simulink model "im_with_m1act_damp"  (R2022b)
settings: Solver=FixedStepAuto  StartTime=0.0  StopTime=5  FixedStep=FEM_Ts  MaxStep=FEM_Ts  RelTol=1e-2
InitFcn:
  | %
  | % Initialization callback function
  | %
  | 
  | try
  |    fprintf('\nGMT IMS version (%s)!\n',simulink_fname );
  | 
  |    % Get Simulink model directory
  |    [filepath,name,ext] = fileparts(which(bdroot));
  | 
  |    if ~strcmp(filepath,pwd)
  |       fprintf('\nChanging current directory to \n %s \n',filepath);
  |       cd(filepath);
  |    end
  | 
  |    %
  |  if(osim.bpless_wl)
  |     fprintf('Generating bumpless wind load time series\n');
  |  end
  | catch
  |    warning('Running the InitFcn from puSimulate script');
  | end
values from neighbouring files (symbols this model uses):
  a_max = 250e-6    (= 0.00025)    [load_im_with_m1act_damp.m]    (also in load_m1hp_cpp_demo.m)
  b = B(:,in)*m1sys{seg}.Kbal    [evalM1ofl_act_damp.m]
  c = [Upsilon*C(out0,:);     C(out1a,:)-C(out1b,:);     C(out2,:)]    [evalM1ofl_act_damp.m]
  CS_Upsilon = [0 0 1 3.6925 1.6038 0 0 0 1 0.99769 3.9002 0 ... (1836 elements, 6x306)]    [CS_SupportActuatorArrayConfig.mat]
  delta_sim = 1e-3    (= 0.001)    [load_im_with_m1act_damp.m]    (also in load_m1hp_cpp_demo.m)
  drv_delay = ceil(mount.delay/FEM_Ts)    [load_im_with_m1act_damp.m]    (also in load_m1hp_cpp_demo.m)
  FEM_Ts = 1/1e3    (= 0.001)    [load_im_with_m1act_damp.m]    (also in load_m1hp_cpp_demo.m)
  Hdrive_d = c2d(o.Hdrive(1,1), FEM_Ts, 'tustin')    [load_im_with_m1act_damp.m]    (also in load_m1hp_cpp_demo.m)
  m1_act_lin_d = osim.m1act_damp*1800    [load_im_with_m1act_damp.m]
  m1_act_quad_d = 9000    [load_im_with_m1act_damp.m]
  m1sys = ovr_ofl_crtl(m1sys,seg)    [evalM1ofl_act_damp.m]    (also in load_im_with_m1act_damp.m = ovr_ofl_crtl(m1sys))
  M_cs_abc2xyz = M_cs_abc2xyzT'    [calc_ort2cylTs.m]
  M_oa_abc2xyz = M_oa_abc2xyzT'    [calc_ort2cylTs.m]
  o = fun_confBase(oTest)    [load_im_with_m1act_damp.m]    (also in load_m1hp_cpp_demo.m)
  OA_Upsilon = [1 0 0 0 -0.308856 0.000749419 0 1 0 0.308856 0 0.776768 ... (2010 elements, 6x335)]    [OA_SupportActuatorArrayConfig.mat]
  PG = zeros(length(om2),6)    [load_im_with_m1act_damp.m]    (also in load_m1hp_cpp_demo.m)
  phiB = inputs2ModalF(mode_ind_vec,indDesInputs)    [load_im_with_m1act_damp.m]    (also in load_m1hp_cpp_demo.m)
  phiC = modalDisp2Outputs(indDesOutputs,mode_ind_vec)    [load_im_with_m1act_damp.m]    (also in load_m1hp_cpp_demo.m)
  phiCvel = modalDisp2Outputs(ind_M1act_vel,mode_ind_vec)    [load_im_with_m1act_damp.m]
  Psi_ss = gainMatrix(indDesOutputs,indDesInputs) - K_ss    [load_im_with_m1act_damp.m]    (also in load_m1hp_cpp_demo.m)
  t_gd = 0*0.5    (= 0)    [load_im_with_m1act_damp.m]    (also in load_m1hp_cpp_demo.m)
  t_gd_v = 0*t_gd    (= 0)    [load_im_with_m1act_damp.m]    (also in load_m1hp_cpp_demo.m)
  Tcmd = 12    [load_im_with_m1act_damp.m]    (also in load_m1hp_cpp_demo.m)
  v0 = 0    [load_im_with_m1act_damp.m]    (also in load_m1hp_cpp_demo.m)
  v_max = 50e-6    (= 5e-05)    [load_im_with_m1act_damp.m]    (also in load_m1hp_cpp_demo.m)
  x0 = 0    [load_im_with_m1act_damp.m]    (also in load_m1hp_cpp_demo.m)
  x0_f = xf(end,:)    [load_im_with_m1act_damp.m]    (also in load_m1hp_cpp_demo.m)
undefined symbols (not defined in the file or in its folder): a, A_f, az, az_ff_en, B_f, C_f, D_f, DiscIntNeverNeededParam, el, gir, M_cs_xyz2abc, M_oa_xyz2abc, magnitude, mount, osim
libraries: simulink x9, ims_block_library x7, simulink_extras x2
(part 2 of 3)

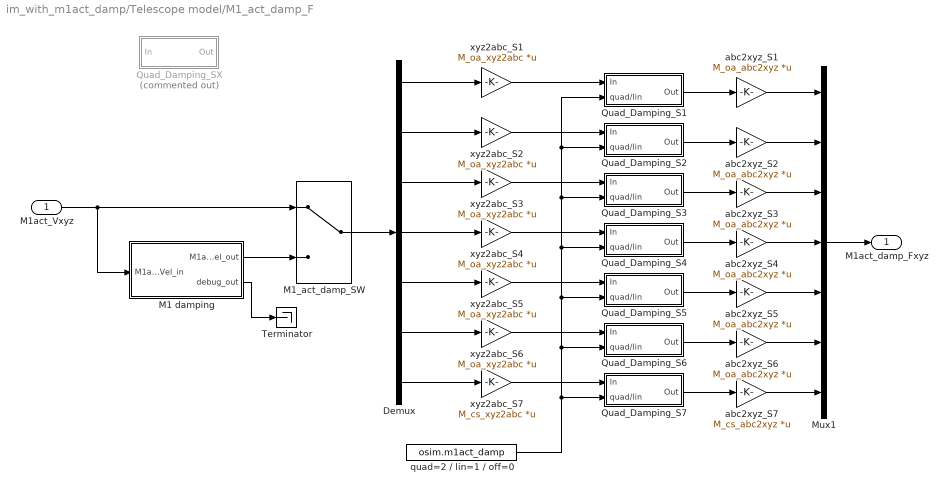
== system im_with_m1act_damp/Telescope model/M1_act_damp_F ==
  M1act_Vxyz : Inport
  Demux : Demux  Outputs=[335,335,335,335,335,335,306]
  M1 damping : Subsystem
  M1_act_damp_SW : ManualSwitch
  Mux1 : Mux  Inputs=[335,335,335,335,335,335,306]
  Quad_Damping_S1 : Subsystem
  Quad_Damping_S2 : Subsystem
  Quad_Damping_S3 : Subsystem
  Quad_Damping_S4 : Subsystem
  Quad_Damping_S5 : Subsystem
  Quad_Damping_S6 : Subsystem
  Quad_Damping_S7 : Subsystem
  Quad_Damping_SX : Subsystem  Commented=on
  Terminator : Terminator
  abc2xyz_S{1..6} (6 alike) : Gain  Gain=M_oa_abc2xyz  Multiplication=Matrix(K*u) (u vector)
  abc2xyz_S7 : Gain  Gain=M_cs_abc2xyz  Multiplication=Matrix(K*u) (u vector)
  quad=2 / lin=1 / off=0 : Constant  Value=osim.m1act_damp
  xyz2abc_S{1..6} (6 alike) : Gain  Gain=M_oa_xyz2abc  Multiplication=Matrix(K*u) (u vector)
  xyz2abc_S7 : Gain  Gain=M_cs_xyz2abc  Multiplication=Matrix(K*u) (u vector)
  M1act_damp_Fxyz : Outport
  wires:
  M1 damping/1(M1act_Vel_out) -> M1_act_damp_SW/2
  Mux1/1 -> M1act_damp_Fxyz/1
  M1act_Vxyz/1 -> M1 damping/1(M1act_Vel_in), M1_act_damp_SW/1
  M1 damping/2(debug_out) -> Terminator/1
  Quad_Damping_S1/1(Out) -> abc2xyz_S1/1
  xyz2abc_S2/1 -> Quad_Damping_S2/1(In)
  abc2xyz_S4/1 -> Mux1/4
  Demux/2 -> xyz2abc_S2/1
  abc2xyz_S7/1 -> Mux1/7
  Demux/5 -> xyz2abc_S5/1
  Quad_Damping_S7/1(Out) -> abc2xyz_S7/1
  Demux/7 -> xyz2abc_S7/1
  abc2xyz_S3/1 -> Mux1/3
  xyz2abc_S5/1 -> Quad_Damping_S5/1(In)
  M1_act_damp_SW/1 -> Demux/1
  Quad_Damping_S6/1(Out) -> abc2xyz_S6/1
  abc2xyz_S1/1 -> Mux1/1
  xyz2abc_S3/1 -> Quad_Damping_S3/1(In)
  Quad_Damping_S5/1(Out) -> abc2xyz_S5/1
  Demux/3 -> xyz2abc_S3/1
  abc2xyz_S2/1 -> Mux1/2
  Quad_Damping_S4/1(Out) -> abc2xyz_S4/1
  Demux/1 -> xyz2abc_S1/1
  xyz2abc_S7/1 -> Quad_Damping_S7/1(In)
  Demux/4 -> xyz2abc_S4/1
  Demux/6 -> xyz2abc_S6/1
  Quad_Damping_S2/1(Out) -> abc2xyz_S2/1
  xyz2abc_S4/1 -> Quad_Damping_S4/1(In)
  xyz2abc_S1/1 -> Quad_Damping_S1/1(In)
  abc2xyz_S6/1 -> Mux1/6
  xyz2abc_S6/1 -> Quad_Damping_S6/1(In)
  Quad_Damping_S3/1(Out) -> abc2xyz_S3/1
  abc2xyz_S5/1 -> Mux1/5
  quad=2 / lin=1 / off=0/1 -> Quad_Damping_S6/2(quad/lin), Quad_Damping_S2/2(quad/lin), Quad_Damping_S1/2(quad/lin), Quad_Damping_S3/2(quad/lin), Quad_Damping_S4/2(quad/lin), Quad_Damping_S5/2(quad/lin), Quad_Damping_S7/2(quad/lin)

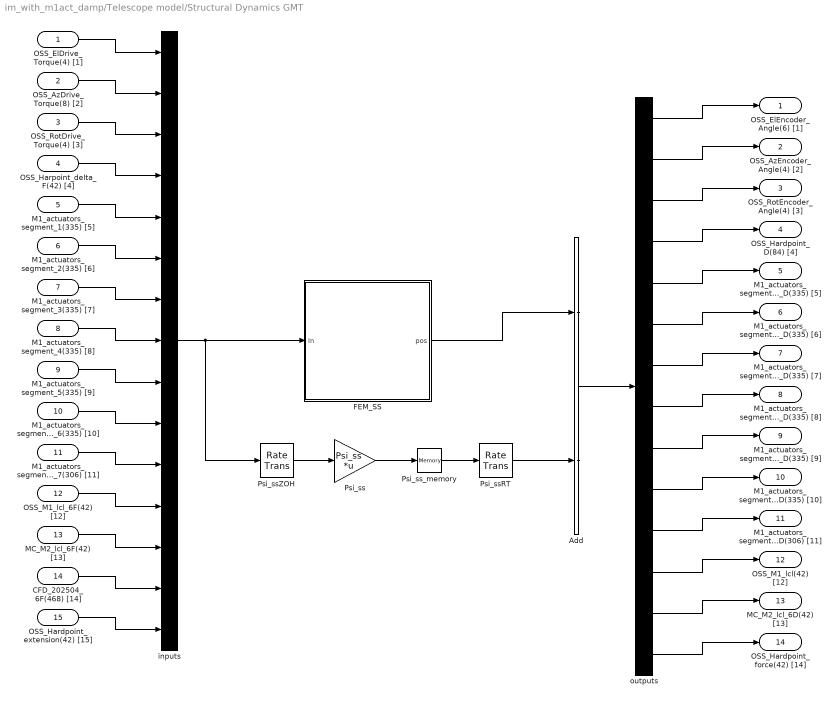
== system im_with_m1act_damp/Telescope model/Structural Dynamics GMT ==
  OSS_ElDrive_Torque(4) [1] : Inport  PortDimensions=4
  OSS_AzDrive_Torque(8) [2] : Inport  Port=2  PortDimensions=8
  OSS_RotDrive_Torque(4) [3] : Inport  Port=3  PortDimensions=4
  OSS_Harpoint_delta_F(42) [4] : Inport  Port=4  PortDimensions=42
  M1_actuators_segment_1(335) [5] : Inport  Port=5  PortDimensions=335
  M1_actuators_segment_2(335) [6] : Inport  Port=6  PortDimensions=335
  M1_actuators_segment_3(335) [7] : Inport  Port=7  PortDimensions=335
  M1_actuators_segment_4(335) [8] : Inport  Port=8  PortDimensions=335
  M1_actuators_segment_5(335) [9] : Inport  Port=9  PortDimensions=335
  M1_actuators_segment_6(335) [10] : Inport  Port=10  PortDimensions=335
  M1_actuators_segment_7(306) [11] : Inport  Port=11  PortDimensions=306
  OSS_M1_lcl_6F(42) [12] : Inport  Port=12  PortDimensions=42
  MC_M2_lcl_6F(42) [13] : Inport  Port=13  PortDimensions=42
  CFD_202504_6F(468) [14] : Inport  Port=14  PortDimensions=468
  OSS_Hardpoint_extension(42) [15] : Inport  Port=15  PortDimensions=42
  Add : Sum
  FEM_SS : Subsystem
  Psi_ss : Gain  Gain=Psi_ss  Multiplication=Matrix(K*u) (u vector)
  Psi_ssRT : RateTransition  Integrity=off  OutPortSampleTimeOpt=Inherit
  Psi_ssZOH : RateTransition  Integrity=off  OutPortSampleTime=Psi_ssTs
  Psi_ss_memory : Memory  InitialCondition=zeros(size(phiC,1),1)  InheritSampleTime=on  LinearizeAsDelay=on
  inputs : Mux  Inputs=modelMuxDims
  outputs : Demux  Outputs=modelDemuxDims
  OSS_ElEncoder_Angle(6) [1] : Outport  PortDimensions=6
  OSS_AzEncoder_Angle(4) [2] : Outport  Port=2  PortDimensions=4
  OSS_RotEncoder_Angle(4) [3] : Outport  Port=3  PortDimensions=4
  OSS_Hardpoint_D(84) [4] : Outport  Port=4  PortDimensions=84
  M1_actuators_segment_1_D(335) [5] : Outport  Port=5  PortDimensions=335
  M1_actuators_segment_2_D(335) [6] : Outport  Port=6  PortDimensions=335
  M1_actuators_segment_3_D(335) [7] : Outport  Port=7  PortDimensions=335
  M1_actuators_segment_4_D(335) [8] : Outport  Port=8  PortDimensions=335
  M1_actuators_segment_5_D(335) [9] : Outport  Port=9  PortDimensions=335
  M1_actuators_segment_6_D(335) [10] : Outport  Port=10  PortDimensions=335
  M1_actuators_segment_7_D(306) [11] : Outport  Port=11  PortDimensions=306
  OSS_M1_lcl(42) [12] : Outport  Port=12  PortDimensions=42
  MC_M2_lcl_6D(42) [13] : Outport  Port=13  PortDimensions=42
  OSS_Hardpoint_force(42) [14] : Outport  Port=14  PortDimensions=42
  wires:
  outputs/14 -> OSS_Hardpoint_force(42) [14]/1
  outputs/13 -> MC_M2_lcl_6D(42) [13]/1
  outputs/12 -> OSS_M1_lcl(42) [12]/1
  outputs/11 -> M1_actuators_segment_7_D(306) [11]/1
  outputs/10 -> M1_actuators_segment_6_D(335) [10]/1
  outputs/9 -> M1_actuators_segment_5_D(335) [9]/1
  outputs/8 -> M1_actuators_segment_4_D(335) [8]/1
  outputs/7 -> M1_actuators_segment_3_D(335) [7]/1
  outputs/6 -> M1_actuators_segment_2_D(335) [6]/1
  outputs/5 -> M1_actuators_segment_1_D(335) [5]/1
  outputs/4 -> OSS_Hardpoint_D(84) [4]/1
  outputs/3 -> OSS_RotEncoder_Angle(4) [3]/1
  outputs/2 -> OSS_AzEncoder_Angle(4) [2]/1
  outputs/1 -> OSS_ElEncoder_Angle(6) [1]/1
  OSS_Hardpoint_extension(42) [15]/1 -> inputs/15
  CFD_202504_6F(468) [14]/1 -> inputs/14
  MC_M2_lcl_6F(42) [13]/1 -> inputs/13
  OSS_M1_lcl_6F(42) [12]/1 -> inputs/12
  M1_actuators_segment_7(306) [11]/1 -> inputs/11
  M1_actuators_segment_6(335) [10]/1 -> inputs/10
  M1_actuators_segment_5(335) [9]/1 -> inputs/9
  M1_actuators_segment_4(335) [8]/1 -> inputs/8
  M1_actuators_segment_3(335) [7]/1 -> inputs/7
  M1_actuators_segment_2(335) [6]/1 -> inputs/6
  M1_actuators_segment_1(335) [5]/1 -> inputs/5
  OSS_Harpoint_delta_F(42) [4]/1 -> inputs/4
  OSS_RotDrive_Torque(4) [3]/1 -> inputs/3
  OSS_AzDrive_Torque(8) [2]/1 -> inputs/2
  OSS_ElDrive_Torque(4) [1]/1 -> inputs/1
  Psi_ssZOH/1 -> Psi_ss/1
  Psi_ss_memory/1 -> Psi_ssRT/1
  Psi_ssRT/1 -> Add/2
  inputs/1 -> Psi_ssZOH/1, FEM_SS/1(In)
  FEM_SS/1(pos) -> Add/1
  Psi_ss/1 -> Psi_ss_memory/1
  Add/1 -> outputs/1

== system im_with_m1act_damp/Wind Loads/Sigmoid ==
  Add : Sum  Inputs=+-
  Add1 : Sum
  Clock : Clock
  Constant : Constant  Value=0.75
  CteOne : Constant
  Gain : Gain  Gain=-5
  Math Function : Math  SignedPower=on
  Reciprocal Function : Math  Operator=reciprocal  SignedPower=on
  Sqr Function : Math  Operator=square  SignedPower=on
  s : Outport
  wires:
  Sqr Function/1 -> Reciprocal Function/1
  Math Function/1 -> Add1/2
  Gain/1 -> Math Function/1
  Add/1 -> Gain/1
  Clock/1 -> Add/1
  Constant/1 -> Add/2
  Add1/1 -> Sqr Function/1
  CteOne/1 -> Add1/1
  Reciprocal Function/1 -> s/1

== system im_with_m1act_damp/M1 CPP/cmd_pre_proc/Bessel filter ==
  pos_vec : Inport  Partition=on  PartitionDimension=1  PartitionWidth=1  PartitionOffset=0
  vel_vec : Inport  Port=2  Partition=on  PartitionDimension=1  PartitionWidth=1  PartitionOffset=0
  acc_vec : Inport  Port=3  Partition=on  PartitionDimension=1  PartitionWidth=1  PartitionOffset=0
  For Each : ForEach  DisableCoverage=on  SpecifiedNumIters=n_in
  Jerk-limitation : Subsystem
  pos_f_vec : Outport  ConcatenationDimension=1
  vel_f_vec : Outport  Port=2  ConcatenationDimension=1
  acc_f_vec : Outport  Port=3  ConcatenationDimension=1
  wires:
  vel_vec/1 -> Jerk-limitation/2(vel)
  Jerk-limitation/3(pos_f) -> pos_f_vec/1
  Jerk-limitation/2(vel_f) -> vel_f_vec/1
  Jerk-limitation/1(acc_f) -> acc_f_vec/1
  pos_vec/1 -> Jerk-limitation/3(pos)
  acc_vec/1 -> Jerk-limitation/1(acc)

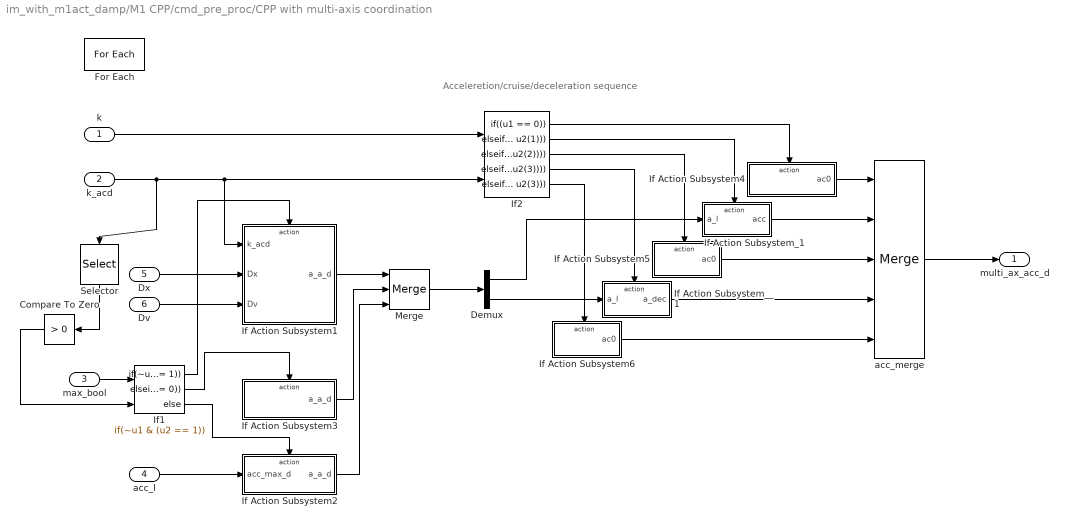
== system im_with_m1act_damp/M1 CPP/cmd_pre_proc/CPP with multi-axis coordination ==
  note: Acceleretion/cruise/deceleration sequence
  k : Inport
  k_acd : Inport  Port=2
  max_bool : Inport  Port=3  Partition=on  PartitionDimension=1  PartitionWidth=1  PartitionOffset=0
  acc_l : Inport  Port=4  Partition=on  PartitionDimension=1  PartitionWidth=1  PartitionOffset=0
  Dx : Inport  Port=5  Partition=on  PartitionDimension=1  PartitionWidth=1  PartitionOffset=0
  Dv : Inport  Port=6  Partition=on  PartitionDimension=1  PartitionWidth=1  PartitionOffset=0
  Compare To Zero : simulink/Logic and Bit Operations/Compare To Zero  relop=>  OutDataTypeStr=boolean
  Demux : Demux  Outputs=2
  For Each : ForEach  DisableCoverage=on
  If Action Subsystem1 : Subsystem  TreatAsAtomicUnit=on
  If Action Subsystem2 : Subsystem  TreatAsAtomicUnit=on
  If Action Subsystem3 : Subsystem  TreatAsAtomicUnit=on
  If Action Subsystem4 : Subsystem  TreatAsAtomicUnit=on
  If Action Subsystem5 : Subsystem  TreatAsAtomicUnit=on
  If Action Subsystem6 : Subsystem  TreatAsAtomicUnit=on
  If Action Subsystem_1 : Subsystem  TreatAsAtomicUnit=on
  If Action Subsystem__1 : Subsystem  TreatAsAtomicUnit=on
  If1 : If  NumInputs=2  IfExpression=~u1 & (u2 == 1)  ElseIfExpressions=~u1 & (u2 == 0)
  If2 : If  NumInputs=2  IfExpression=(u1 == 0)  ElseIfExpressions=(u1 <= u2(1)), ((u1 > u2(1)) & (u1 <= u2(2))), ((u1 > u2(2)) & (u1 <= u2(3))), (u1 > u2(3))  ShowElse=off
  Merge : Merge  Inputs=3
  Selector : Selector  InputPortWidth=3  IndexOptions=Index vector (dialog)  Indices=[3]  OutputSizes=1
  acc_merge : Merge  Inputs=5  InitialOutput=0
  multi_ax_acc_d : Outport  ConcatenationDimension=1
  wires:
  acc_merge/1 -> multi_ax_acc_d/1
  k/1 -> If2/1
  max_bool/1 -> If1/1
  If1/1 -> If Action Subsystem1/Action
  If1/3 -> If Action Subsystem2/Action
  acc_l/1 -> If Action Subsystem2/1(acc_max_d)
  If Action Subsystem2/1(a_a_d) -> Merge/3
  If Action Subsystem1/1(a_a_d) -> Merge/1
  Merge/1 -> Demux/1
  Dx/1 -> If Action Subsystem1/2(Dx)
  Dv/1 -> If Action Subsystem1/3(Dv)
  If Action Subsystem3/1(a_a_d) -> Merge/2
  Selector/1 -> Compare To Zero/1
  If1/2 -> If Action Subsystem3/Action
  Compare To Zero/1 -> If1/2
  If Action Subsystem5/1(ac0) -> acc_merge/3
  If2/1 -> If Action Subsystem4/Action
  Demux/2 -> If Action Subsystem__1/1(a_l)
  If Action Subsystem4/1(ac0) -> acc_merge/1
  If2/3 -> If Action Subsystem5/Action
  If2/4 -> If Action Subsystem__1/Action
  If Action Subsystem__1/1(a_dec) -> acc_merge/4
  If2/2 -> If Action Subsystem_1/Action
  If Action Subsystem_1/1(acc) -> acc_merge/2
  Demux/1 -> If Action Subsystem_1/1(a_l)
  If2/5 -> If Action Subsystem6/Action
  If Action Subsystem6/1(ac0) -> acc_merge/5
  k_acd/1 -> If2/2, If Action Subsystem1/1(k_acd), Selector/1

== system im_with_m1act_damp/M1 CPP/cmd_pre_proc/CPP with multi-axis coordination1 ==
  k : Inport
  k_acd : Inport  Port=2
  Demux1 : Demux  Outputs=3
  Dk_merge : Merge  Inputs=4  InitialOutput=0
  If Action Subsystem : Subsystem  TreatAsAtomicUnit=on
  If Action Subsystem1 : Subsystem  TreatAsAtomicUnit=on
  If Action Subsystem6 : Subsystem  TreatAsAtomicUnit=on
  If Action Subsystem__1 : Subsystem  TreatAsAtomicUnit=on
  If2 : If  NumInputs=2  IfExpression=(u1 == 0) | (u1 <= u2(1))  ElseIfExpressions=((u1 > u2(1)) & (u1 <= u2(2))), ((u1 > u2(2)) & (u1 <= u2(3))), (u1 > u2(3))  ShowElse=off
  Dk : Outport
  wires:
  k_acd/1 -> If2/2, Demux1/1
  k/1 -> If2/1
  Demux1/3 -> If Action Subsystem6/1(t_acd)
  If Action Subsystem__1/1(Dk) -> Dk_merge/3
  Demux1/1 -> If Action Subsystem1/1(t_a)
  If2/1 -> If Action Subsystem/Action
  If Action Subsystem/1(Dk) -> Dk_merge/1
  Demux1/2 -> If Action Subsystem__1/1(t_ac)
  If Action Subsystem1/1(Dk) -> Dk_merge/2
  If Action Subsystem6/1(Dk) -> Dk_merge/4
  Dk_merge/1 -> Dk/1
  If2/2 -> If Action Subsystem1/Action
  If2/3 -> If Action Subsystem__1/Action
  If2/4 -> If Action Subsystem6/Action

== system im_with_m1act_damp/M1 CPP/cmd_pre_proc/Motion equations ==
  acc_d : Inport  Partition=on  PartitionDimension=1  PartitionWidth=1  PartitionOffset=0
  k : Inport  Port=2
  Dk : Inport  Port=3
  Add : Sum  Inputs=+++
  Compare To Constant : simulink/Logic and Bit Operations/Compare To Constant  relop===  const=0  OutDataTypeStr=boolean
  Constant : Constant  Value=v0
  Detect Change : simulink/Logic and Bit Operations/Detect Change  vinit=0  OutDataTypeStr=boolean
  Discrete-Time Integrator : DiscreteIntegrator  IntegratorMethod=Integration: Backward Euler  InitialConditionSource=external  InitialCondition=v0  SampleTime=-1  ICPrevOutput=DiscIntNeverNeededParam  ICPrevScaledInput=DiscIntNeverNeededParam
  For Each : ForEach  DisableCoverage=on
  Gain : Gain  Gain=0.5
  Gain1 : Gain  Gain=delta_sim  OutDataTypeStr=double
  Logical Operator : Logic  Operator=OR  IconShape=distinctive  AllPortsSameDT=off  OutDataTypeStr=boolean
  Math Function : Math  Operator=magnitude^2
  Product : Product
  Product1 : Product
  Subtract1 : Sum  Inputs=+-
  Triggered Subsystem : Subsystem  TreatAsAtomicUnit=on
  pos_d_vec : Outport  ConcatenationDimension=1
  vel_d_vec : Outport  Port=2  ConcatenationDimension=1
  wires:
  Detect Change/1 -> Logical Operator/1
  Add/1 -> pos_d_vec/1, Triggered Subsystem/1(x0_in)
  [x0] -> Add/3
  Gain/1 -> Product/1
  Constant/1 -> Discrete-Time Integrator/2
  Math Function/1 -> Product/2
  Triggered Subsystem/2(v0) -> Product1/2
  Product/1 -> Add/1
  acc_d/1 -> Discrete-Time Integrator/1, Gain/1, Detect Change/1
  Triggered Subsystem/1(x0) -> [x0]
  Discrete-Time Integrator/1 -> vel_d_vec/1, Triggered Subsystem/2(v0_in)
  Product1/1 -> Add/2
  k/1 -> Subtract1/1, Compare To Constant/1
  Gain1/1 -> Product1/1, Math Function/1
  Subtract1/1 -> Gain1/1
  Logical Operator/1 -> Triggered Subsystem/Trigger
  Compare To Constant/1 -> Logical Operator/2
  Dk/1 -> Subtract1/2

== system im_with_m1act_damp/M1 CPP/cmd_pre_proc/Sample_generator ==
  Add : Sum
  Compare To Constant : simulink/Logic and Bit Operations/Compare To Constant  relop===  const=floor(Tcmd/delta_sim)  OutDataTypeStr=boolean
  Constant : Constant  OutDataTypeStr=uint32
  Resettable Delay : Delay  DelayLength=1  ExternalReset=Rising
      settings: InputPortMap=u0,r5
  Unit Delay : UnitDelay  SampleTime=-1  HasFrameUpgradeWarning=on
  k : Outport
  wires:
  Constant/1 -> Add/1
  Add/1 -> Resettable Delay/1, Unit Delay/1
  Resettable Delay/1 -> k/1, Add/2
  Compare To Constant/1 -> Resettable Delay/2
  Unit Delay/1 -> Compare To Constant/1

== system im_with_m1act_damp/M1 CPP/cmd_pre_proc/Triggered Subsystem ==
  x1_multi_ax : Inport
  x0_multi_ax : Inport  Port=2  LatchByDelayingOutsideSignal=on
  v0_multi_ax : Inport  Port=3  LatchByDelayingOutsideSignal=on
  v1_multi_ax : Inport  Port=4
  Trigger : TriggerPort  VariantControl=Variant  InitialTriggerSignalState=zero
  Add : Sum  Inputs=+-
  Detect max t_seg : Subsystem
  Detect max t_seg_varsize : Subsystem  Commented=on
  Display : Display  Commented=on
  Display t_seg : Display  Commented=on
  Index Vector : MultiPortSwitch  Inputs=1  RndMeth=Simplest  SaturateOnIntegerOverflow=off
  Index Vector1 : MultiPortSwitch  Inputs=1  RndMeth=Simplest  SaturateOnIntegerOverflow=off
  Index Vector2 : MultiPortSwitch  Inputs=1  RndMeth=Simplest  SaturateOnIntegerOverflow=off
  Multi-axis demand : Subsystem  TreatAsAtomicUnit=on
  Mux : Mux  Inputs=3
  Sub : Sum  Inputs=+-
  k_a_ac_acd : Outport
  max_bool : Outport  Port=2
  a_l : Outport  Port=3
  Dx : Outport  Port=4
  Dv : Outport  Port=5
  wires:
  x1_multi_ax/1 -> Add/1, Multi-axis demand/1(x1)
  x0_multi_ax/1 -> Add/2, Multi-axis demand/2(x0)
  Detect max t_seg/1(max_idx) -> Index Vector1/1, Index Vector/1, Index Vector2/1
  v0_multi_ax/1 -> Sub/2, Multi-axis demand/4(v0)
  v1_multi_ax/1 -> Sub/1, Multi-axis demand/3(v1)
  Multi-axis demand/3(t_a_d) -> Index Vector/2, Display t_seg/1, Detect max t_seg/1(t_seg)
  Multi-axis demand/4(a_l) -> a_l/1
  Multi-axis demand/1(t_a) -> Index Vector2/2
  Multi-axis demand/2(t_a_c) -> Index Vector1/2
  Index Vector2/1 -> Mux/1
  Index Vector1/1 -> Mux/2
  Index Vector/1 -> Mux/3
  Mux/1 -> k_a_ac_acd/1, Display/1
  Add/1 -> Dx/1
  Sub/1 -> Dv/1
  Detect max t_seg/2(max_bool) -> max_bool/1

== system im_with_m1act_damp/Mount_Drv_FDR2023_linear/DRV Friction/AZ DT Lugre Fr mode ==
  v : Inport
  Enable : EnablePort
  Constant : Constant  Value=iIsSig01Active
  Discrete-Time Integrator : DiscreteIntegrator  SampleTime=-1  ICPrevOutput=DiscIntNeverNeededParam  ICPrevScaledInput=DiscIntNeverNeededParam
  Sum : Sum  Inputs=+++
  g(v) : Subsystem
  sigma_0 : Gain  Gain=sigma0
  sigma_1 : Gain  Gain=sigma1
  sigma_v : Gain  Gain=sigmav
  v2z : Subsystem
  Tfr : Outport
  wires:
  Constant/1 -> g(v)/Enable, v2z/Enable
  v/1 -> sigma_v/1, v2z/1(v), g(v)/1(v)
  sigma_v/1 -> Sum/3
  sigma_1/1 -> Sum/1
  Sum/1 -> Tfr/1
  sigma_0/1 -> Sum/2
  g(v)/1(g) -> v2z/2(g(v))
  Discrete-Time Integrator/1 -> v2z/3(z), sigma_0/1
  v2z/1(dz) -> sigma_1/1, Discrete-Time Integrator/1

== system im_with_m1act_damp/Mount_Drv_FDR2023_linear/DRV Friction/EL DT Lugre Fr model ==
  v : Inport
  Enable : EnablePort
  Constant : Constant  Value=iIsSig01Active
  Discrete-Time Integrator : DiscreteIntegrator  SampleTime=-1  ICPrevOutput=DiscIntNeverNeededParam  ICPrevScaledInput=DiscIntNeverNeededParam
  Sum : Sum  Inputs=+++
  g(v) : Subsystem
  sigma_0 : Gain  Gain=sigma0
  sigma_1 : Gain  Gain=sigma1
  sigma_v : Gain  Gain=sigmav
  v2z : Subsystem
  Tfr : Outport
  wires:
  Constant/1 -> g(v)/Enable, v2z/Enable
  sigma_0/1 -> Sum/2
  Discrete-Time Integrator/1 -> v2z/3(z), sigma_0/1
  g(v)/1(g) -> v2z/2(g(v))
  v/1 -> sigma_v/1, v2z/1(v), g(v)/1(v)
  Sum/1 -> Tfr/1
  sigma_1/1 -> Sum/1
  v2z/1(dz) -> sigma_1/1, Discrete-Time Integrator/1
  sigma_v/1 -> Sum/3

== system im_with_m1act_damp/Mount_Drv_FDR2023_linear/DRV Friction/EL DT Lugre Fr model_ ==
  vel : Inport
  Enable : EnablePort
  Constant : Constant  Value=frParStruct.iIsSig01Active
  Discrete-Time Integrator : DiscreteIntegrator  SampleTime=-1  ICPrevOutput=DiscIntNeverNeededParam  ICPrevScaledInput=DiscIntNeverNeededParam
  Sum : Sum  Inputs=+++
  To Workspace : ToWorkspace  VariableName=el_Ve  SampleTime=-1
  To Workspace1 : ToWorkspace  VariableName=el_To  SampleTime=-1
  g(v) : Subsystem
  sigma_0 : Gain  Gain=frParStruct.sigm0
  sigma_1 : Gain  Gain=frParStruct.sigm1
  sigma_v : Gain  Gain=frParStruct.sigmv
  v2z : Subsystem
  FrTorque : Outport  VectorParamsAs1DForOutWhenUnconnected=off
  wires:
  Sum/1 -> FrTorque/1, To Workspace1/1
  v2z/1(dz) -> sigma_1/1, Discrete-Time Integrator/1
  Discrete-Time Integrator/1 -> v2z/3(z), sigma_0/1
  sigma_1/1 -> Sum/1
  g(v)/1(g) -> v2z/2(g(v))
  sigma_0/1 -> Sum/2
  Constant/1 -> v2z/Enable, g(v)/Enable
  vel/1 -> sigma_v/1, To Workspace/1, g(v)/1(v), v2z/1(v)
  sigma_v/1 -> Sum/3  "Viscose Friction"

== system im_with_m1act_damp/Mount_Drv_FDR2023_linear/DRV Friction/GIR DT Lugre Fr model ==
  note: Discretized blocks
  v : Inport
  Enable : EnablePort
  Discrete Transfer Fcn : DiscreteTransferFcn  Numerator=[1 1]  Denominator="[1+(1/pi/20/FEM_Ts),  (1-(1/pi/20/FEM_Ts))]"  SampleTime=FEM_Ts
  Discrete-Time Integrator : DiscreteIntegrator  SampleTime=FEM_Ts  ICPrevOutput=DiscIntNeverNeededParam  ICPrevScaledInput=DiscIntNeverNeededParam
  Sum : Sum  Inputs=+++
  g(v) : Subsystem
  iIsSig01Active : Gain  Gain=iIsSig01Active
  on/off : Gain
  sigma_0 : Gain  Gain=sigma0
  sigma_1 : Gain  Gain=sigma1
  sigma_v : Gain  Gain=sigmav
  v2z : Subsystem
      settings: MinAlgLoopOccurrences=on
  Tfr : Outport
  wires:
  Discrete Transfer Fcn/1 -> sigma_1/1
  on/off/1 -> Sum/1
  sigma_1/1 -> on/off/1
  Sum/1 -> Tfr/1
  v/1 -> sigma_v/1, iIsSig01Active/1
  iIsSig01Active/1 -> v2z/1(v), g(v)/1(v)
  sigma_v/1 -> Sum/3
  sigma_0/1 -> Sum/2
  Discrete-Time Integrator/1 -> v2z/3(z), sigma_0/1
  v2z/1(dz) -> Discrete Transfer Fcn/1, Discrete-Time Integrator/1
  g(v)/1(g) -> v2z/2(g(v))

== system im_with_m1act_damp/Mount_Drv_FDR2023_linear/DRV Friction/GIR DT Lugre Fr model_ ==
  vel : Inport
  Enable : EnablePort
  Discrete-Time Integrator : DiscreteIntegrator  SampleTime=-1  ICPrevOutput=DiscIntNeverNeededParam  ICPrevScaledInput=DiscIntNeverNeededParam
  Gain : Gain  Gain=frParStruct.iIsSig01Active
  Scope : Scope  Commented=on  NumInputPorts=2
  Scope1 : Scope  NumInputPorts=3
  Sum : Sum  Inputs=+++
  To Workspace : ToWorkspace  VariableName=gir_Ve  SampleTime=-1
  To Workspace1 : ToWorkspace  VariableName=gir_To  SampleTime=-1
  g(v) : Subsystem
  sigma_0 : Gain  Gain=frParStruct.sigm0
  sigma_1 : Gain  Gain=frParStruct.sigm1
  sigma_v : Gain  Gain=frParStruct.sigmv
  v2z : Subsystem
  FrTorque : Outport  VectorParamsAs1DForOutWhenUnconnected=off
  wires:
  sigma_1/1 -> Sum/1, Scope1/1  "sigma1*dz"
  sigma_0/1 -> Sum/2, Scope1/2  "sigma0*z"
  Gain/1 -> g(v)/1(v), v2z/1(v)
  Sum/1 -> FrTorque/1, To Workspace1/1
  v2z/1(dz) -> Scope/1, sigma_1/1, Discrete-Time Integrator/1  "dz"
  Discrete-Time Integrator/1 -> v2z/3(z), sigma_0/1, Scope/2  "z"
  g(v)/1(g) -> v2z/2(g(v))
  vel/1 -> sigma_v/1, To Workspace/1, Gain/1
  sigma_v/1 -> Sum/3, Scope1/3  "Viscous Friction"

== system im_with_m1act_damp/Mount_Drv_FDR2023_linear/Friction/Friction Alt ==
  v : Inport
  Enable : EnablePort
  Constant : Constant  Value=iIsSig01Active
  Integrator2 : Integrator
  Sum : Sum  Inputs=+++
  g(v) : Subsystem
  sigma_0 : Gain  Gain=sigma0
  sigma_1 : Gain  Gain=sigma1
  sigma_v : Gain  Gain=sigmav
  v2z : Subsystem
  Tfr : Outport
  wires:
  v2z/1(dz) -> Integrator2/1, sigma_1/1
  Integrator2/1 -> sigma_0/1, v2z/3(z)
  g(v)/1(g) -> v2z/2(g(v))
  sigma_0/1 -> Sum/2
  Sum/1 -> Tfr/1
  sigma_1/1 -> Sum/1
  sigma_v/1 -> Sum/3
  v/1 -> g(v)/1(v), v2z/1(v), sigma_v/1
  Constant/1 -> v2z/Enable, g(v)/Enable

== system im_with_m1act_damp/Mount_Drv_FDR2023_linear/Friction/Friction Az ==
  v : Inport
  Enable : EnablePort
  Constant : Constant  Value=iIsSig01Active
  Integrator2 : Integrator
  Sum : Sum  Inputs=+++
  g(v) : Subsystem
  sigma_0 : Gain  Gain=sigma0
  sigma_1 : Gain  Gain=sigma1
  sigma_v : Gain  Gain=sigmav
  v2z : Subsystem
  Tfr : Outport
  wires:
  v2z/1(dz) -> Integrator2/1, sigma_1/1
  Integrator2/1 -> sigma_0/1, v2z/3(z)
  g(v)/1(g) -> v2z/2(g(v))
  sigma_0/1 -> Sum/2
  Sum/1 -> Tfr/1
  sigma_1/1 -> Sum/1
  sigma_v/1 -> Sum/3
  v/1 -> g(v)/1(v), v2z/1(v), sigma_v/1
  Constant/1 -> g(v)/Enable, v2z/Enable

== system im_with_m1act_damp/Mount_Drv_FDR2023_linear/Friction/Friction Gir ==
  v : Inport
  Enable : EnablePort
  Integrator2 : Integrator
  PT1 : Subsystem  mask{f=20}
      mask prompts: f "f(Hz)"
      mask Display: fprintf('PT1')
  Sum : Sum  Inputs=+++
  g(v) : Subsystem
  iIsSig01Active : Gain  Gain=iIsSig01Active
  on/off : Gain
  sigma_0 : Gain  Gain=sigma0
  sigma_1 : Gain  Gain=sigma1
  sigma_v : Gain  Gain=sigmav
  v2z : Subsystem
      settings: MinAlgLoopOccurrences=on
  Tfr : Outport
  wires:
  g(v)/1(g) -> v2z/2(g(v))
  v2z/1(dz) -> PT1/1(in), Integrator2/1
  Integrator2/1 -> sigma_0/1, v2z/3(z)
  sigma_0/1 -> Sum/2
  sigma_v/1 -> Sum/3
  iIsSig01Active/1 -> g(v)/1(v), v2z/1(v)
  v/1 -> iIsSig01Active/1, sigma_v/1
  Sum/1 -> Tfr/1
  sigma_1/1 -> on/off/1
  on/off/1 -> Sum/1
  PT1/1(out) -> sigma_1/1

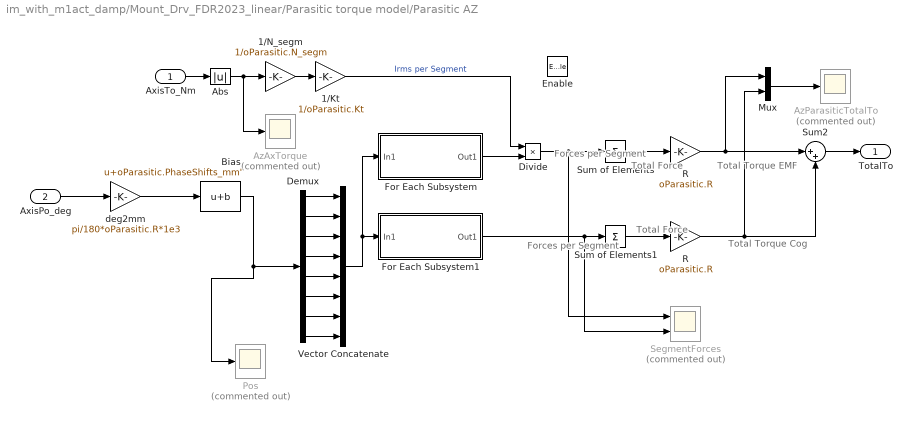
== system im_with_m1act_damp/Mount_Drv_FDR2023_linear/Parasitic torque model/Parasitic AZ ==
  note: Total
      | Torque Cog
  note: Total
      | Torque EMF
  note: Total
      | Force
  note: Forces per
      | Segment
  note: Forces per
      | Segment
  note: Total
      | Force
  AxisTo_Nm : Inport
  AxisPo_deg : Inport  Port=2
  Enable : EnablePort
  1/Kt : Gain  Gain=1/oParasitic.Kt
  1/N_segm : Gain  Gain=1/oParasitic.N_segm
  Abs : Abs  SaturateOnIntegerOverflow=off
  AzAxTorque : Scope  Commented=on
  AzParasiticTotalTo : Scope  Commented=on
  Bias : Bias  Bias=oParasitic.PhaseShifts_mm'  SaturateOnIntegerOverflow=off
  Demux : Demux  Outputs=8
  Divide : Product  Inputs=**
  For Each Subsystem : Subsystem  TreatAsAtomicUnit=on
  For Each Subsystem1 : Subsystem  TreatAsAtomicUnit=on
  Mux : Mux  Inputs=2
  Pos : Scope  Commented=on
  R : Gain  Gain=oParasitic.R
  "R " : Gain  Gain=oParasitic.R
  SegmentForces : Scope  Commented=on  NumInputPorts=2
  Sum of Elements : Sum  Inputs=+
  Sum of Elements1 : Sum  Inputs=+
  Sum2 : Sum  Inputs=|++
  Vector Concatenate : Concatenate  NumInputs=oParasitic.N_segm
  deg2mm : Gain  Gain=pi/180*oParasitic.R*1e3
  TotalTo : Outport
  wires:
  AxisPo_deg/1 -> deg2mm/1
  deg2mm/1 -> Bias/1
  Abs/1 -> 1/N_segm/1, AzAxTorque/1
  AxisTo_Nm/1 -> Abs/1
  Demux/8 -> Vector Concatenate/8
  Demux/7 -> Vector Concatenate/7
  Demux/6 -> Vector Concatenate/6
  Demux/5 -> Vector Concatenate/5
  Demux/4 -> Vector Concatenate/4
  Demux/3 -> Vector Concatenate/3
  Demux/2 -> Vector Concatenate/2
  Demux/1 -> Vector Concatenate/1
  For Each Subsystem1/1(Out1) -> Sum of Elements1/1, SegmentForces/2
  For Each Subsystem/1(Out1) -> Divide/2
  Vector Concatenate/1 -> For Each Subsystem1/1(In1), For Each Subsystem/1(In1)
  Bias/1 -> Pos/1, Demux/1
  Mux/1 -> AzParasiticTotalTo/1
  1/Kt/1 -> Divide/1  "Irms per Segment"
  Sum of Elements/1 -> R/1
  1/N_segm/1 -> 1/Kt/1
  R/1 -> Sum2/1, Mux/1
  "R "/1 -> Mux/2, Sum2/2
  Divide/1 -> SegmentForces/1, Sum of Elements/1
  Sum2/1 -> TotalTo/1
  Sum of Elements1/1 -> "R "/1

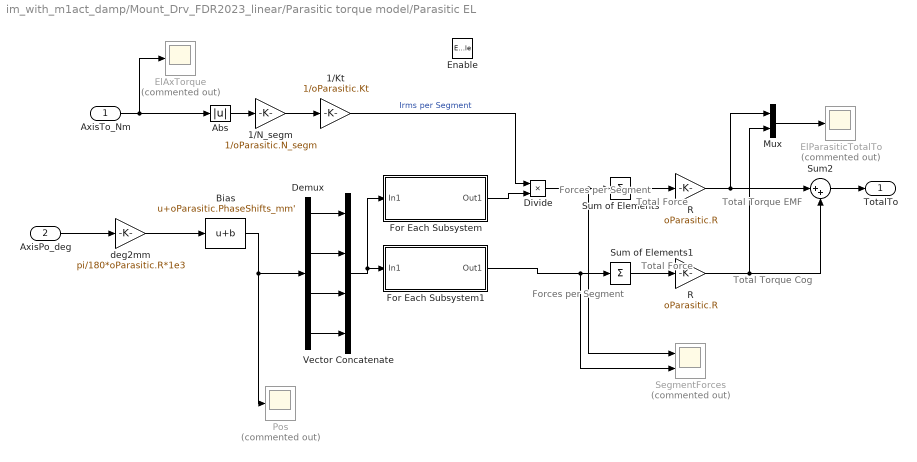
== system im_with_m1act_damp/Mount_Drv_FDR2023_linear/Parasitic torque model/Parasitic EL ==
  note: Total
      | Torque Cog
  note: Total
      | Torque EMF
  note: Total
      | Force
  note: Forces per
      | Segment
  note: Forces per
      | Segment
  note: Total
      | Force
  AxisTo_Nm : Inport
  AxisPo_deg : Inport  Port=2
  Enable : EnablePort
  1/Kt : Gain  Gain=1/oParasitic.Kt
  1/N_segm : Gain  Gain=1/oParasitic.N_segm
  Abs : Abs  SaturateOnIntegerOverflow=off
  Bias : Bias  Bias=oParasitic.PhaseShifts_mm'  SaturateOnIntegerOverflow=off
  Demux : Demux  Outputs=oParasitic.N_segm
  Divide : Product  Inputs=**
  ElAxTorque : Scope  Commented=on
  ElParasiticTotalTo : Scope  Commented=on
  For Each Subsystem : Subsystem  TreatAsAtomicUnit=on
  For Each Subsystem1 : Subsystem  TreatAsAtomicUnit=on
  Mux : Mux  Inputs=2
  Pos : Scope  Commented=on
  R : Gain  Gain=oParasitic.R
  "R " : Gain  Gain=oParasitic.R
  SegmentForces : Scope  Commented=on  NumInputPorts=2
  Sum of Elements : Sum  Inputs=+
  Sum of Elements1 : Sum  Inputs=+
  Sum2 : Sum  Inputs=|++
  Vector Concatenate : Concatenate  NumInputs=oParasitic.N_segm
  deg2mm : Gain  Gain=pi/180*oParasitic.R*1e3
  TotalTo : Outport
  wires:
  AxisPo_deg/1 -> deg2mm/1
  deg2mm/1 -> Bias/1
  Abs/1 -> 1/N_segm/1
  AxisTo_Nm/1 -> Abs/1, ElAxTorque/1
  Demux/4 -> Vector Concatenate/4
  Demux/3 -> Vector Concatenate/3
  Demux/2 -> Vector Concatenate/2
  Demux/1 -> Vector Concatenate/1
  For Each Subsystem1/1(Out1) -> Sum of Elements1/1, SegmentForces/2
  For Each Subsystem/1(Out1) -> Divide/2
  Vector Concatenate/1 -> For Each Subsystem1/1(In1), For Each Subsystem/1(In1)
  Bias/1 -> Demux/1, Pos/1
  Mux/1 -> ElParasiticTotalTo/1
  1/Kt/1 -> Divide/1  "Irms per Segment"
  Sum of Elements/1 -> R/1
  1/N_segm/1 -> 1/Kt/1
  R/1 -> Sum2/1, Mux/1
  "R "/1 -> Mux/2, Sum2/2
  Divide/1 -> SegmentForces/1, Sum of Elements/1
  Sum2/1 -> TotalTo/1
  Sum of Elements1/1 -> "R "/1

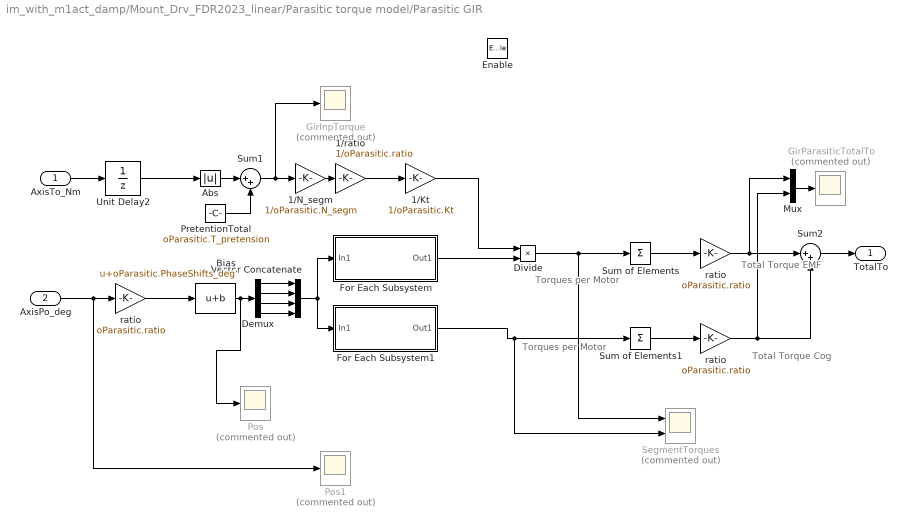
== system im_with_m1act_damp/Mount_Drv_FDR2023_linear/Parasitic torque model/Parasitic GIR ==
  note: Total
      | Torque Cog
  note: Total
      | Torque EMF
  note: Torques
      | per Motor
  note: Torques per
      | Motor
  AxisTo_Nm : Inport
  AxisPo_deg : Inport  Port=2
  Enable : EnablePort
  1/Kt : Gain  Gain=1/oParasitic.Kt
  1/N_segm : Gain  Gain=1/oParasitic.N_segm
  "1/ratio   " : Gain  Gain=1/oParasitic.ratio
  Abs : Abs  SaturateOnIntegerOverflow=off
  Bias : Bias  Bias=oParasitic.PhaseShifts_deg'  SaturateOnIntegerOverflow=off
  Demux : Demux
  Divide : Product  Inputs=**
  For Each Subsystem : Subsystem  TreatAsAtomicUnit=on
  For Each Subsystem1 : Subsystem  TreatAsAtomicUnit=on
  GirInpTorque : Scope  Commented=on
  GirParasiticTotalTo : Scope  Commented=on
  Mux : Mux  Inputs=2
  Pos : Scope  Commented=on
  Pos1 : Scope  Commented=on
  PretentionTotal : Constant  Value=oParasitic.T_pretension
  SegmentTorques : Scope  Commented=on  NumInputPorts=2
  Sum of Elements : Sum  Inputs=+
  Sum of Elements1 : Sum  Inputs=+
  Sum1 : Sum  Inputs=|++
  Sum2 : Sum  Inputs=|++
  Unit Delay2 : UnitDelay  SampleTime=-1  HasFrameUpgradeWarning=on
  Vector Concatenate : Concatenate  NumInputs=oParasitic.N_segm
  ratio : Gain  Gain=oParasitic.ratio
  "ratio " : Gain  Gain=oParasitic.ratio
  "ratio  " : Gain  Gain=oParasitic.ratio
  TotalTo : Outport
  wires:
  Unit Delay2/1 -> Abs/1
  AxisTo_Nm/1 -> Unit Delay2/1
  Sum1/1 -> 1/N_segm/1, GirInpTorque/1
  1/Kt/1 -> Divide/1
  PretentionTotal/1 -> Sum1/2
  Abs/1 -> Sum1/1
  "1/ratio   "/1 -> 1/Kt/1
  1/N_segm/1 -> "1/ratio   "/1
  Bias/1 -> Demux/1, Pos/1
  Demux/4 -> Vector Concatenate/4
  Demux/3 -> Vector Concatenate/3
  Demux/2 -> Vector Concatenate/2
  Demux/1 -> Vector Concatenate/1
  Vector Concatenate/1 -> For Each Subsystem1/1(In1), For Each Subsystem/1(In1)
  For Each Subsystem/1(Out1) -> Divide/2
  For Each Subsystem1/1(Out1) -> Sum of Elements1/1, SegmentTorques/2
  "ratio  "/1 -> Sum2/1, Mux/1
  "ratio "/1 -> Mux/2, Sum2/2
  Sum of Elements/1 -> "ratio  "/1
  Sum of Elements1/1 -> "ratio "/1
  ratio/1 -> Bias/1
  AxisPo_deg/1 -> ratio/1, Pos1/1
  Mux/1 -> GirParasiticTotalTo/1
  Divide/1 -> Sum of Elements/1, SegmentTorques/1
  Sum2/1 -> TotalTo/1

== system im_with_m1act_damp/Mount_Drv_FDR2023_linear/ToothContact Torques/ToothContact GIR (Norm) ==
  AxisPos_deg : Inport
  AxisTo : Inport  Port=2
  1-D Lookup Table : Lookup_n-D  NumberOfTableDimensions=1  BreakpointsForDimension1=oToothContact.oInterp.Pos  Table=oToothContact.oInterp.TorqueRate  InternalRulePriority=Speed  RndMeth=Simplest
  Abs : Abs  SaturateOnIntegerOverflow=off
  Gain : Gain  Gain=0.25
  Max Position : Constant  Value=oToothContact.maxPos
  Phase Shifts : Constant  Value=oToothContact.PhaseShift_deg
  PretensionTotal : Constant  Value=gir.T_pretension
  Product1 : Product  RndMeth=Zero
  Rem : Math  Operator=rem
  Sum of Elements : Sum  Inputs=+  CollapseMode=Specified dimension
  Sum1 : Sum  Inputs=|++
  Sum2 : Sum  Inputs=|++
  TotalTo : Outport
  wires:
  AxisTo/1 -> Abs/1
  Gain/1 -> Product1/2
  Sum1/1 -> Gain/1
  PretensionTotal/1 -> Sum1/2
  Abs/1 -> Sum1/1
  AxisPos_deg/1 -> Sum2/1
  Sum of Elements/1 -> TotalTo/1
  Phase Shifts/1 -> Sum2/2
  Sum2/1 -> Rem/1
  1-D Lookup Table/1 -> Product1/1
  Rem/1 -> 1-D Lookup Table/1
  Max Position/1 -> Rem/2
  Product1/1 -> Sum of Elements/1  "Position"

== system im_with_m1act_damp/Mount_Drv_FDR2023_linear/ToothContact Torques/ToothContact GIR (Peak) ==
  AxisPos_deg : Inport
  AxisTo : Inport  Port=2
  1-D Lookup Table : Lookup_n-D  NumberOfTableDimensions=1  BreakpointsForDimension1=oToothContact.oInterp.Pos  Table=oToothContact.oInterp.TorqueRate  InternalRulePriority=Speed  RndMeth=Simplest
  Abs : Abs  SaturateOnIntegerOverflow=off
  Gain : Gain  Gain=0.25
  Max Position : Constant  Value=oToothContact.maxPos
  Phase Shifts : Constant  Value=oToothContact.PhaseShift_deg
  PretensionTotal : Constant  Value=gir.T_pretension
  Product1 : Product  RndMeth=Zero
  Rem : Math  Operator=rem
  Sum of Elements : Sum  Inputs=+  CollapseMode=Specified dimension
  Sum1 : Sum  Inputs=|++
  Sum2 : Sum  Inputs=|++
  TotalTo : Outport
  wires:
  AxisTo/1 -> Abs/1
  Gain/1 -> Product1/2
  Sum1/1 -> Gain/1
  PretensionTotal/1 -> Sum1/2
  Abs/1 -> Sum1/1
  AxisPos_deg/1 -> Sum2/1
  Sum of Elements/1 -> TotalTo/1
  Phase Shifts/1 -> Sum2/2
  Sum2/1 -> Rem/1
  1-D Lookup Table/1 -> Product1/1
  Rem/1 -> 1-D Lookup Table/1
  Max Position/1 -> Rem/2
  Product1/1 -> Sum of Elements/1  "Position"

== system im_with_m1act_damp/Telescope model/M1_act_damp_F/M1 damping ==
  M1act_Vel_in : Inport
  Demux : Demux  Outputs=[335,335,335,335,335,335,306]
  Force balance S1 : Gain  Gain=m1sys{1}.Kbal  Multiplication=Matrix(K*u)
  Force balance S2 : Gain  Gain=m1sys{2}.Kbal  Multiplication=Matrix(K*u)
  Force balance S3 : Gain  Gain=m1sys{3}.Kbal  Multiplication=Matrix(K*u)
  Force balance S4 : Gain  Gain=m1sys{4}.Kbal  Multiplication=Matrix(K*u)
  Force balance S5 : Gain  Gain=m1sys{5}.Kbal  Multiplication=Matrix(K*u)
  Force balance S6 : Gain  Gain=m1sys{6}.Kbal  Multiplication=Matrix(K*u)
  Force balance S7 : Gain  Gain=m1sys{7}.Kbal  Multiplication=Matrix(K*u)
  Mux1 : Mux  Inputs=[335,335,335,335,335,335,306]
  Upsilon{1..6} (6 alike) : Gain  Gain=OA_Upsilon  Multiplication=Matrix(K*u)
  Upsilon7 : Gain  Gain=CS_Upsilon  Multiplication=Matrix(K*u)
  M1act_Vel_out : Outport
  debug_out : Outport  Port=2
  wires:
  Mux1/1 -> M1act_Vel_out/1
  M1act_Vel_in/1 -> Demux/1
  Demux/1 -> Upsilon1/1
  Demux/2 -> Upsilon2/1
  Demux/3 -> Upsilon3/1
  Demux/4 -> Upsilon4/1
  Demux/5 -> Upsilon5/1
  Demux/6 -> Upsilon6/1
  Demux/7 -> Upsilon7/1
  Upsilon7/1 -> debug_out/1, Force balance S7/1
  Upsilon6/1 -> Force balance S6/1
  Upsilon5/1 -> Force balance S5/1
  Upsilon4/1 -> Force balance S4/1
  Upsilon3/1 -> Force balance S3/1
  Upsilon2/1 -> Force balance S2/1
  Upsilon1/1 -> Force balance S1/1
  Force balance S1/1 -> Mux1/1
  Force balance S2/1 -> Mux1/2
  Force balance S3/1 -> Mux1/3
  Force balance S4/1 -> Mux1/4
  Force balance S5/1 -> Mux1/5
  Force balance S6/1 -> Mux1/6
  Force balance S7/1 -> Mux1/7

== system im_with_m1act_damp/Telescope model/M1_act_damp_F/Quad_Damping_S1 ==
  In : Inport
  quad/lin : Inport  Port=2
  Abs : Abs  SaturateOnIntegerOverflow=off
  Math Function : Math  Operator=square
  Product : Product
  Sign : Signum
  Switch : Switch  Criteria=u2 > Threshold  Threshold=1  SaturateOnIntegerOverflow=off  InputSameDT=off
  lin_damp : Gain  Gain=m1_act_lin_d
  quad_damp : Gain  Gain=m1_act_quad_d
  Out : Outport
  wires:
  Math Function/1 -> quad_damp/1
  In/1 -> Abs/1, Sign/1, Math Function/1
  Sign/1 -> Product/1
  Product/1 -> Out/1
  Abs/1 -> lin_damp/1
  quad_damp/1 -> Switch/1
  lin_damp/1 -> Switch/3
  Switch/1 -> Product/2
  quad/lin/1 -> Switch/2

== system im_with_m1act_damp/Telescope model/M1_act_damp_F/Quad_Damping_S2 ==
  In : Inport
  quad/lin : Inport  Port=2
  Abs : Abs  SaturateOnIntegerOverflow=off
  Math Function : Math  Operator=square
  Product : Product
  Sign : Signum
  Switch : Switch  Criteria=u2 > Threshold  Threshold=1  SaturateOnIntegerOverflow=off  InputSameDT=off
  lin_damp : Gain  Gain=m1_act_lin_d
  quad_damp : Gain  Gain=m1_act_quad_d
  Out : Outport
  wires:
  Math Function/1 -> quad_damp/1
  In/1 -> Abs/1, Sign/1, Math Function/1
  Sign/1 -> Product/1
  Product/1 -> Out/1
  Abs/1 -> lin_damp/1
  quad_damp/1 -> Switch/1
  lin_damp/1 -> Switch/3
  Switch/1 -> Product/2
  quad/lin/1 -> Switch/2

== system im_with_m1act_damp/Telescope model/M1_act_damp_F/Quad_Damping_S3 ==
  In : Inport
  quad/lin : Inport  Port=2
  Abs : Abs  SaturateOnIntegerOverflow=off
  Math Function : Math  Operator=square
  Product : Product
  Sign : Signum
  Switch : Switch  Criteria=u2 > Threshold  Threshold=1  SaturateOnIntegerOverflow=off  InputSameDT=off
  lin_damp : Gain  Gain=m1_act_lin_d
  quad_damp : Gain  Gain=m1_act_quad_d
  Out : Outport
  wires:
  Math Function/1 -> quad_damp/1
  In/1 -> Abs/1, Sign/1, Math Function/1
  Sign/1 -> Product/1
  Product/1 -> Out/1
  Abs/1 -> lin_damp/1
  quad_damp/1 -> Switch/1
  lin_damp/1 -> Switch/3
  Switch/1 -> Product/2
  quad/lin/1 -> Switch/2

== system im_with_m1act_damp/Telescope model/M1_act_damp_F/Quad_Damping_S4 ==
  In : Inport
  quad/lin : Inport  Port=2
  Abs : Abs  SaturateOnIntegerOverflow=off
  Math Function : Math  Operator=square
  Product : Product
  Sign : Signum
  Switch : Switch  Criteria=u2 > Threshold  Threshold=1  SaturateOnIntegerOverflow=off  InputSameDT=off
  lin_damp : Gain  Gain=m1_act_lin_d
  quad_damp : Gain  Gain=m1_act_quad_d
  Out : Outport
  wires:
  Math Function/1 -> quad_damp/1
  In/1 -> Abs/1, Sign/1, Math Function/1
  Sign/1 -> Product/1
  Product/1 -> Out/1
  Abs/1 -> lin_damp/1
  quad_damp/1 -> Switch/1
  lin_damp/1 -> Switch/3
  Switch/1 -> Product/2
  quad/lin/1 -> Switch/2

== system im_with_m1act_damp/Telescope model/M1_act_damp_F/Quad_Damping_S5 ==
  In : Inport
  quad/lin : Inport  Port=2
  Abs : Abs  SaturateOnIntegerOverflow=off
  Math Function : Math  Operator=square
  Product : Product
  Sign : Signum
  Switch : Switch  Criteria=u2 > Threshold  Threshold=1  SaturateOnIntegerOverflow=off  InputSameDT=off
  lin_damp : Gain  Gain=m1_act_lin_d
  quad_damp : Gain  Gain=m1_act_quad_d
  Out : Outport
  wires:
  Math Function/1 -> quad_damp/1
  In/1 -> Abs/1, Sign/1, Math Function/1
  Sign/1 -> Product/1
  Product/1 -> Out/1
  Abs/1 -> lin_damp/1
  quad_damp/1 -> Switch/1
  lin_damp/1 -> Switch/3
  Switch/1 -> Product/2
  quad/lin/1 -> Switch/2

== system im_with_m1act_damp/Telescope model/M1_act_damp_F/Quad_Damping_S6 ==
  In : Inport
  quad/lin : Inport  Port=2
  Abs : Abs  SaturateOnIntegerOverflow=off
  Math Function : Math  Operator=square
  Product : Product
  Sign : Signum
  Switch : Switch  Criteria=u2 > Threshold  Threshold=1  SaturateOnIntegerOverflow=off  InputSameDT=off
  lin_damp : Gain  Gain=m1_act_lin_d
  quad_damp : Gain  Gain=m1_act_quad_d
  Out : Outport
  wires:
  Math Function/1 -> quad_damp/1
  In/1 -> Abs/1, Sign/1, Math Function/1
  Sign/1 -> Product/1
  Product/1 -> Out/1
  Abs/1 -> lin_damp/1
  quad_damp/1 -> Switch/1
  lin_damp/1 -> Switch/3
  Switch/1 -> Product/2
  quad/lin/1 -> Switch/2

== system im_with_m1act_damp/Telescope model/M1_act_damp_F/Quad_Damping_S7 ==
  In : Inport
  quad/lin : Inport  Port=2
  Abs : Abs  SaturateOnIntegerOverflow=off
  Math Function : Math  Operator=square
  Product : Product
  Sign : Signum
  Switch : Switch  Criteria=u2 > Threshold  Threshold=1  SaturateOnIntegerOverflow=off  InputSameDT=off
  lin_damp : Gain  Gain=m1_act_lin_d
  quad_damp : Gain  Gain=m1_act_quad_d
  Out : Outport
  wires:
  Math Function/1 -> quad_damp/1
  In/1 -> Abs/1, Sign/1, Math Function/1
  Sign/1 -> Product/1
  Product/1 -> Out/1
  Abs/1 -> lin_damp/1
  quad_damp/1 -> Switch/1
  lin_damp/1 -> Switch/3
  Switch/1 -> Product/2
  quad/lin/1 -> Switch/2

== system im_with_m1act_damp/Telescope model/M1_act_damp_F/Quad_Damping_SX ==
  In : Inport
  Constant : Constant
  Math Function : Math  Commented=through  Operator=square
  Product : Product
  Sign : Signum  Commented=on
  quad_damp : Gain  Gain=m1_act_lin_d%m1_act_quad_d
  Out : Outport
  wires:
  Math Function/1 -> quad_damp/1
  In/1 -> Sign/1, Math Function/1
  quad_damp/1 -> Product/2
  Product/1 -> Out/1
  Constant/1 -> Product/1

== system im_with_m1act_damp/Telescope model/Structural Dynamics GMT/FEM_SS ==
  note: 2nd order form simulation
  In : Inport
  Sum2 : Sum  Inputs=+++
  Sum3 : Sum  Inputs=+++
  Unit Delay : UnitDelay  SampleTime=FEM_Ts  HasFrameUpgradeWarning=on
  Unit Delay1 : UnitDelay  SampleTime=FEM_Ts  HasFrameUpgradeWarning=on
  gamma1 : Gain  Gain=PG(:,3)
  gamma2 : Gain  Gain=PG(:,6)
  phi11 : Gain  Gain=PG(:,1)
  phi12 : Gain  Gain=PG(:,2)
  phi21 : Gain  Gain=PG(:,4)
  phi22 : Gain  Gain=PG(:,5)
  phiB : Gain  Gain=phiB  Multiplication=Matrix(K*u) (u vector)
  phiC : Gain  Gain=phiC  Multiplication=Matrix(K*u) (u vector)
  phiCvel : Gain  Commented=on  Gain=phiCvel  Multiplication=Matrix(K*u) (u vector)
  pos : Outport  VectorParamsAs1DForOutWhenUnconnected=off
  wires:
  Unit Delay/1 -> phi11/1, phi21/1, phiC/1
  phi12/1 -> Sum3/2
  Sum2/1 -> Unit Delay1/1
  Sum3/1 -> Unit Delay/1
  gamma2/1 -> Sum2/3
  phi21/1 -> Sum2/2
  phi22/1 -> Sum2/1
  gamma1/1 -> Sum3/1
  phi11/1 -> Sum3/3
  phiB/1 -> gamma2/1, gamma1/1
  phiC/1 -> pos/1
  In/1 -> phiB/1
  Unit Delay1/1 -> phiCvel/1, phi12/1, phi22/1

== system im_with_m1act_damp/M1 CPP/cmd_pre_proc/Bessel filter/Jerk-limitation ==
  acc : Inport
  vel : Inport  Port=2
  pos : Inport  Port=3
  Add1 : Sum  Inputs=+++
  Add2 : Sum
  Bessel filter Acc : DiscreteStateSpace  A=A_f  B=B_f  C=C_f  D=D_f  InitialCondition=x0_f * 0  SampleTime=delta_sim
  Bessel filter Pos : DiscreteStateSpace  A=A_f  B=B_f  C=C_f  D=D_f  InitialCondition=x0_f * x0  SampleTime=delta_sim
  Bessel filter Vel : DiscreteStateSpace  A=A_f  B=B_f  C=C_f  D=D_f  InitialCondition=x0_f * v0  SampleTime=delta_sim
  Gain1 : Gain  Gain=t_gd
  Gain2 : Gain  Gain=t_gd_v
  Gain3 : Gain  Gain=t_gd^2
  acc_f : Outport
  vel_f : Outport  Port=2
  pos_f : Outport  Port=3
  wires:
  pos/1 -> Add1/2
  Bessel filter Pos/1 -> pos_f/1
  Bessel filter Acc/1 -> acc_f/1
  vel/1 -> Add2/2, Gain1/1
  Add2/1 -> Bessel filter Vel/1
  acc/1 -> Gain3/1, Bessel filter Acc/1, Gain2/1
  Bessel filter Vel/1 -> vel_f/1
  Gain2/1 -> Add2/1
  Gain1/1 -> Add1/1
  Gain3/1 -> Add1/3
  Add1/1 -> Bessel filter Pos/1

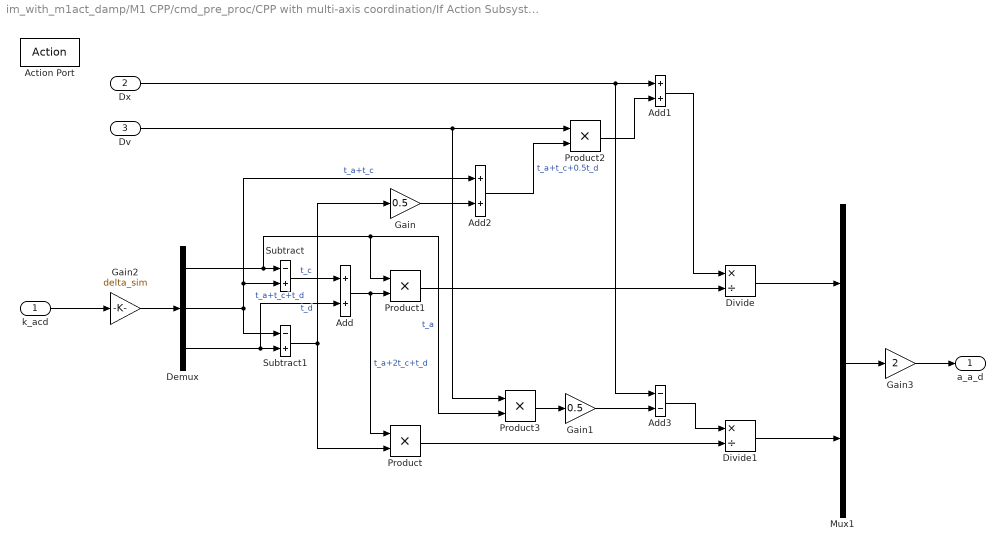
== system im_with_m1act_damp/M1 CPP/cmd_pre_proc/CPP with multi-axis coordination/If Action Subsystem1 ==
  k_acd : Inport
  Dx : Inport  Port=2
  Dv : Inport  Port=3
  Action Port : ActionPort  ActionPortLabel=if(~u1 & (u2 == 1))
  Add : Sum
  Add1 : Sum
  Add2 : Sum
  Add3 : Sum  Inputs=--
  Demux : Demux  Outputs=3
  Divide : Product  Inputs=*/
  Divide1 : Product  Inputs=*/
  Gain : Gain  Gain=0.5
  Gain1 : Gain  Gain=0.5
  Gain2 : Gain  Gain=delta_sim  OutDataTypeStr=double
  Gain3 : Gain  Gain=2
  Mux1 : Mux  Inputs=2
  Product{,1..3} (4 alike) : Product
  Subtract : Sum  Inputs=-+
  Subtract1 : Sum  Inputs=-+
  a_a_d : Outport
  wires:
  Gain3/1 -> a_a_d/1
  Divide1/1 -> Mux1/2
  Demux/3 -> Add/2, Subtract1/2  "t_a+t_c+t_d"
  Add2/1 -> Product2/2  "t_a+t_c+0.5t_d"
  Gain1/1 -> Add3/2
  Product2/1 -> Add1/2
  Divide/1 -> Mux1/1
  Add3/1 -> Divide1/1
  Mux1/1 -> Gain3/1
  Product3/1 -> Gain1/1
  Product/1 -> Divide1/2
  Subtract/1 -> Add/1  "t_c"
  Dv/1 -> Product3/1, Product2/1
  Dx/1 -> Add3/1, Add1/1
  Add/1 -> Product/1, Product1/2  "t_a+2t_c+t_d"
  Demux/1 -> Product3/2, Product1/1, Subtract/1  "t_a"
  Product1/1 -> Divide/2
  Gain/1 -> Add2/2
  Subtract1/1 -> Gain/1, Product/2  "t_d"
  Demux/2 -> Subtract1/1, Add2/1, Subtract/2  "t_a+t_c"
  Add1/1 -> Divide/1
  k_acd/1 -> Gain2/1
  Gain2/1 -> Demux/1

== system im_with_m1act_damp/M1 CPP/cmd_pre_proc/CPP with multi-axis coordination/If Action Subsystem2 ==
  acc_max_d : Inport
  Action Port : ActionPort  ActionPortLabel=else
  Mux : Mux  Inputs=2
  Unary Minus : UnaryMinus
  a_a_d : Outport
  wires:
  acc_max_d/1 -> Unary Minus/1, Mux/1
  Mux/1 -> a_a_d/1
  Unary Minus/1 -> Mux/2

== system im_with_m1act_damp/M1 CPP/cmd_pre_proc/CPP with multi-axis coordination/If Action Subsystem3 ==
  Action Port : ActionPort  ActionPortLabel=elseif(~u1 & (u2 == 0))
  Constant : Constant  Value=0
  Mux : Mux  Inputs=2
  a_a_d : Outport
  wires:
  Mux/1 -> a_a_d/1
  Constant/1 -> Mux/2, Mux/1

== system im_with_m1act_damp/M1 CPP/cmd_pre_proc/CPP with multi-axis coordination/If Action Subsystem4 ==
  Action Port : ActionPort  ActionPortLabel=if((u1 == 0))
  Constant : Constant  Value=0
  ac0 : Outport  VectorParamsAs1DForOutWhenUnconnected=off
  wires:
  Constant/1 -> ac0/1

== system im_with_m1act_damp/M1 CPP/cmd_pre_proc/CPP with multi-axis coordination/If Action Subsystem5 ==
  Action Port : ActionPort  ActionPortLabel=elseif( ((u1 > u2(1)) & (u1 <= u2(2))))
  Constant : Constant  Value=0
  ac0 : Outport  VectorParamsAs1DForOutWhenUnconnected=off
  wires:
  Constant/1 -> ac0/1

== system im_with_m1act_damp/M1 CPP/cmd_pre_proc/CPP with multi-axis coordination/If Action Subsystem6 ==
  Action Port : ActionPort  ActionPortLabel=elseif( (u1 > u2(3)))
  Constant : Constant  Value=0
  ac0 : Outport  VectorParamsAs1DForOutWhenUnconnected=off
  wires:
  Constant/1 -> ac0/1

== system im_with_m1act_damp/M1 CPP/cmd_pre_proc/CPP with multi-axis coordination/If Action Subsystem_1 ==
  a_l : Inport
  Action Port : ActionPort  ActionPortLabel=elseif((u1 <= u2(1)))
  acc : Outport  InitialOutput=0  VectorParamsAs1DForOutWhenUnconnected=off
  wires:
  a_l/1 -> acc/1

== system im_with_m1act_damp/M1 CPP/cmd_pre_proc/CPP with multi-axis coordination/If Action Subsystem__1 ==
  a_l : Inport
  Action Port : ActionPort  ActionPortLabel=elseif( ((u1 > u2(2)) & (u1 <= u2(3))))
  a_dec : Outport  InitialOutput=0  VectorParamsAs1DForOutWhenUnconnected=off
  wires:
  a_l/1 -> a_dec/1

== system im_with_m1act_damp/M1 CPP/cmd_pre_proc/CPP with multi-axis coordination1/If Action Subsystem ==
  Action Port : ActionPort  ActionPortLabel=if((u1 == 0) | (u1 <= u2(1)))
  Constant1 : Constant  Value=0  OutDataTypeStr=uint32
  Dk : Outport  VectorParamsAs1DForOutWhenUnconnected=off
  wires:
  Constant1/1 -> Dk/1

== system im_with_m1act_damp/M1 CPP/cmd_pre_proc/CPP with multi-axis coordination1/If Action Subsystem1 ==
  t_a : Inport
  Action Port : ActionPort  ActionPortLabel=elseif(((u1 > u2(1)) & (u1 <= u2(2))))
  Dk : Outport  InitialOutput=0  VectorParamsAs1DForOutWhenUnconnected=off
  wires:
  t_a/1 -> Dk/1

== system im_with_m1act_damp/M1 CPP/cmd_pre_proc/CPP with multi-axis coordination1/If Action Subsystem6 ==
  t_acd : Inport
  Action Port : ActionPort  ActionPortLabel=elseif( (u1 > u2(3)))
  Dk : Outport  InitialOutput=0  VectorParamsAs1DForOutWhenUnconnected=off
  wires:
  t_acd/1 -> Dk/1

== system im_with_m1act_damp/M1 CPP/cmd_pre_proc/CPP with multi-axis coordination1/If Action Subsystem__1 ==
  t_ac : Inport
  Action Port : ActionPort  ActionPortLabel=elseif( ((u1 > u2(2)) & (u1 <= u2(3))))
  Dk : Outport  InitialOutput=0  VectorParamsAs1DForOutWhenUnconnected=off
  wires:
  t_ac/1 -> Dk/1

== system im_with_m1act_damp/M1 CPP/cmd_pre_proc/Motion equations/Triggered Subsystem ==
  x0_in : Inport  LatchByDelayingOutsideSignal=on
  v0_in : Inport  Port=2  LatchByDelayingOutsideSignal=on
  Trigger : TriggerPort  VariantControl=Variant
  x0 : Outport  SourceOfInitialOutputValue=Input signal  InitialOutput=[x0]  VectorParamsAs1DForOutWhenUnconnected=off
  v0 : Outport  Port=2  InitialOutput=[v0]  VectorParamsAs1DForOutWhenUnconnected=off
  wires:
  x0_in/1 -> x0/1
  v0_in/1 -> v0/1
